simulink model "docexconnectionlabel"  (R2022a)
settings: Solver=FixedStepAuto  StartTime=0.0  StopTime=0  RelTol=1e-3  EnableMultiTasking=on
values from neighbouring files (symbols this model uses):
  x = [3 1]    [CreateVirtualConnectionsUsingConnectionLabelBlockExample.m]    (also in input.mat = [3 2])
undefined symbols (not defined in the file or in its folder): magnitude
libraries: simrfV2util1 x3, simrfV2sources1 x1, simrfV2elements x1
settings Model: Creator=The MathWorks, Inc.  LastModifiedBy=zg88
settings SolverCC: AlgebraicLoopSolver=TrustRegion  MaxZcPerStep=1
settings DataIOCC: LimitDataPoints=on  SaveOutput=off  SignalLogging=off  DSMLogging=off  SaveTime=off
settings OptimizationCC: ExpressionDepthLimit=2147483647  LifeSpan=inf
settings DebuggingCC: UnderspecifiedInitializationDetection=Classic  MergeDetectMultiDrivingBlocksExec=none  SolverPrmCheckMsg=warning  UnconnectedInputMsg=warning  UnconnectedOutputMsg=warning  UnconnectedLineMsg=warning  StateNameClashWarn=warning  SFUnexpectedBacktrackingDiag=warning  SFNoUnconditionalDefaultTransitionDiag=warning  SFExecutionAtInitializationDiag=none  SFMachineParentedDataDiag=warning  ArithmeticOperatorsInVariantConditions=warning
settings HardwareCC: ProdBitPerPointer=32  ProdBitPerSizeT=32  ProdBitPerPtrDiffT=32  ProdLargestAtomicFloat=None  ProdIntDivRoundTo=Undefined  ProdEndianess=Unspecified  ProdWordSize=32  ProdHWDeviceType=32-bit Generic
settings ModelReferenceCC: PropagateSignalLabelsOutOfModel=off
settings SFSimCC: SimUseLocalCustomCode=off  CustomCodeUndefinedFunction=UseInterfaceOnly
settings RTWCC: RTWUseLocalCustomCode=off  DLArmComputeVersion=19.05
settings CodeAppCC: StateflowObjectComments=on
settings GRTTargetCC: TargetLangStandard=C89/C90 (ANSI)
settings ConfigComp: CovMetricSettings=dw  CovSaveCumulativeToWorkspaceVar=on  CovSaveSingleToWorkspaceVar=on  CovExternalEMLEnable=off
settings SimscapeCC: SimscapeNormalizeSystem=off  SimscapeNominalValues="[{\"value\":\"10\",\"unit\":\"V\"},{\"value\":\"1\",\"unit\":\"A\"},{\"value\":\"10\",\"unit\":\"N*m\"},{\"value\":\"10\",\"unit\":\"bar\"},{\"value\":\"100\",\"unit\":\"kJ/kg\"},{\"value\":\"1\",\"unit\":\"kW\"},{\"value\":\"300\",\"unit\":\"K\"},{\"value\":\"100\",\"unit\":\"cm^3/s\"},{\"value\":\"1\",\"unit\":\"kN\"},{\"value\":\"1\",\"unit\":\"g/cm^3\"},{\"value\":\"1\",\"unit\":\"l\"},{\"value\":\"1\",\"unit\":\"cm^2\"},{\"value\":\"60\",\"unit\":\"Hz\"}]"

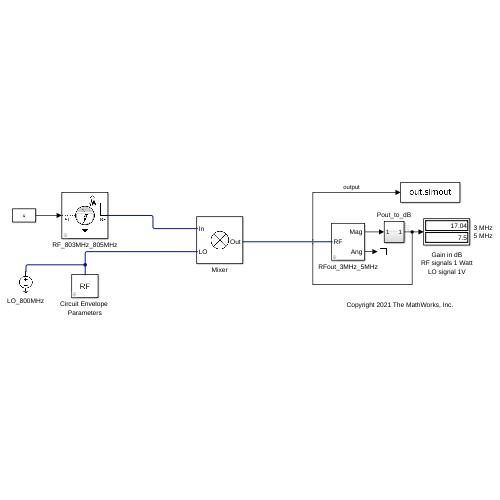
[thumbnail: Simulink's stored preview of the top-level diagram]
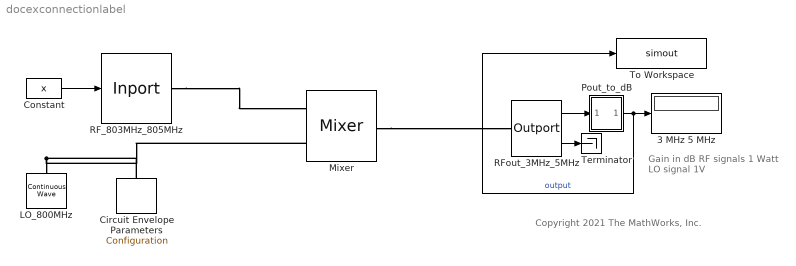
== system docexconnectionlabel ==
  note: Gain in dB
      | RF signals 1 Watt
      | LO signal 1V
  note: Copyright 2021 The MathWorks, Inc.
  3 MHz 5 MHz : Display
  Circuit Envelope Parameters : simrfV2util1/Configuration  AutoFreq=off  Tones="[800  1] MHz"  Harmonics="[1      5]"  NormalizeCarrierPower=off  SolverType=Auto  UseCCode=on  StepSize=1e-7 s  AddNoise=off  defaultRNG=on  Seed=0  Temperature=290 K  SolverDelFlag=0  AbsTol=1e-6  RelTol=1e-3  MaxIter=10  ErrorEstimationType=2-norm over all variables  EnableInterpFilter=off  HiddenFIRfilterControllerParam=on  SmallSignalApprox=off  AllSimFreqs=on  SimFreqs=[] Hz  SimFreqsInternal=[]  SamplesPerFrame=1
      settings: SourceProductBaseCode=RB
  Constant : Constant  Value=x
  LO_800MHz : simrfV2sources1/Continuous Wave  CWSourceType=Ideal voltage  Z0=0  IVoltage=1 V  ICurrent=0 A  MagPower=1/sqrt(2) W  QVoltage=0 V  QCurrent=0 A  AnglePower=0  CarrierFreq=800 MHz  AddPhaseNoise=off  PhaseNoiseOffset=1  PhaseNoiseLevel=-Inf  AutoImpulseLength=on  ImpulseLength=1e-10 s  InternalGrounding=on
      settings: SourceProductBaseCode=RB
  Mixer : simrfV2elements/Mixer  classname=mixer  Source_linear_gain=Available power gain  linear_gain=7.5 dB  Zin=50  Zout=50  ZLO=inf  Source_Poly=Odd order  Poly_Coeffs=[0 1]  IPType=Output  IP2=Inf dBm  IP3=Inf dBm  P1dB=Inf dBm  Psat=inf dBm  Gcomp=Inf dBm  NF=0  InternalGrounding=on
      settings: SourceProductBaseCode=RB
  Pout_to_dB : Subsystem
  RF_803MHz_805MHz : simrfV2util1/Inport  SimulinkInputSignalType=Power  CarrierFreq=[803 805] MHz  ZS=50  InternalGrounding=on
      settings: SourceProductBaseCode=RB
  RFout_3MHz_5MHz : simrfV2util1/Outport  SensorType=Power  OutputFormat=Magnitude and Angle Baseband  CarrierFreq=[3 5] MHz  ZL=50  InternalGrounding=on  StepSize=-1 s  AutoStep=off
      settings: SourceProductBaseCode=RB
  Terminator : Terminator
  To Workspace : ToWorkspace  VariableName=simout  SaveFormat=Timeseries  SampleTime=-1
  wires:
  RFout_3MHz_5MHz/1 -> Pout_to_dB/1(In1)
  Constant/1 -> RF_803MHz_805MHz/1
  RFout_3MHz_5MHz/2 -> Terminator/1
  Pout_to_dB/1(Out1) -> To Workspace/1, 3 MHz 5 MHz/1  "output"
  connections:
  Mixer/RConn1 -- RFout_3MHz_5MHz/LConn1
  LO_800MHz/LConn1 -- Mixer/LConn2 -- Circuit Envelope Parameters/LConn1
  RF_803MHz_805MHz/RConn1 -- Mixer/LConn1

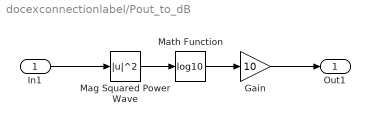
== system docexconnectionlabel/Pout_to_dB ==
  In1 : Inport
  Gain : Gain  Gain=10
  Mag Squared Power Wave : Math  Operator=magnitude^2
  Math Function : Math  Operator=log10
  Out1 : Outport
  wires:
  Math Function/1 -> Gain/1
  Mag Squared Power Wave/1 -> Math Function/1
  Gain/1 -> Out1/1
  In1/1 -> Mag Squared Power Wave/1
